simulink model "V4_Modell_komplett"  (R2022a)
settings: Solver=ode3  StartTime=0.0  StopTime=Zeit(end)  FixedStep=0.00001  RelTol=1e-3
values from neighbouring files (symbols this model uses):
  A = 0.01155    [V4_Parameter_Wagen_St.m]    (also in V4_Parameter_Wagen_Te.m; V4_Parameter_komplett_St.m; V4_Parameter_komplett_Te.m)
  c_W = 0.81    [V4_Parameter_Wagen_St.m]    (also in V4_Parameter_Wagen_Te.m; V4_Parameter_komplett_St.m; V4_Parameter_komplett_Te.m)
  g = 9.81    [V4_Parameter_Wagen_St.m]    (also in V4_Parameter_Wagen_Te.m; V4_Parameter_komplett_St.m; V4_Parameter_komplett_Te.m)
  gamma_rad = gamma_deg * (pi/180)    (= 0.349065850399)    [V4_Parameter_Wagen_St.m]    (also in V4_Parameter_Wagen_Te.m; V4_Parameter_komplett_St.m; V4_Parameter_komplett_Te.m)
  k = (m_Trans + m_ErsatzAntrieb + m_ErsatzRad) / (m_Trans)    [V4_Parameter_Wagen_St.m]    (also in V4_Parameter_Wagen_Te.m; V4_Parameter_komplett_St.m; V4_Parameter_komplett_Te.m)
  k_M = -0.038462    [V4_Parameter_EM.m]    (also in V4_Parameter_Wagen_St.m; V4_Parameter_Wagen_Te.m; V4_Parameter_komplett_St.m; V4_Parameter_komplett_Te.m)
  KL_R_VH = [10      20      30      40 ... (first row only)    [V4_Parameter_EM.m]    (also in V4_Parameter_komplett_St.m; V4_Parameter_komplett_Te.m)
  L_A = 0.11 * (10^(-3))    (= 0.00011)    [V4_Parameter_EM.m]    (also in V4_Parameter_komplett_St.m; V4_Parameter_komplett_Te.m)
  m_Trans = m_W + 4*m_R    (= 2.157)    [V4_Parameter_Wagen_St.m]    (also in V4_Parameter_Wagen_Te.m = 1.7232; V4_Parameter_komplett_St.m; V4_Parameter_komplett_Te.m = 1.7232)
  mu_R = 0.043    [V4_Parameter_Wagen_St.m]    (also in V4_Parameter_Wagen_Te.m = 0.045; V4_Parameter_komplett_St.m; V4_Parameter_komplett_Te.m = 0.045)
  R_A = 0.36    [V4_Parameter_EM.m]    (also in V4_Parameter_komplett_St.m; V4_Parameter_komplett_Te.m)
  r_ZR = 25 * (10^(-3))    (= 0.025)    [V4_Parameter_EM.m]    (also in V4_Parameter_Wagen_St.m = 0.021; V4_Parameter_Wagen_Te.m = 0.021; V4_Parameter_komplett_St.m; V4_Parameter_komplett_Te.m)
  rho_L = 1.2    [V4_Parameter_Wagen_St.m]    (also in V4_Parameter_Wagen_Te.m; V4_Parameter_komplett_St.m; V4_Parameter_komplett_Te.m)
undefined symbols (not defined in the file or in its folder): v_rot, x_rot
settings Model: Creator=bornk  LastModifiedBy=bornk

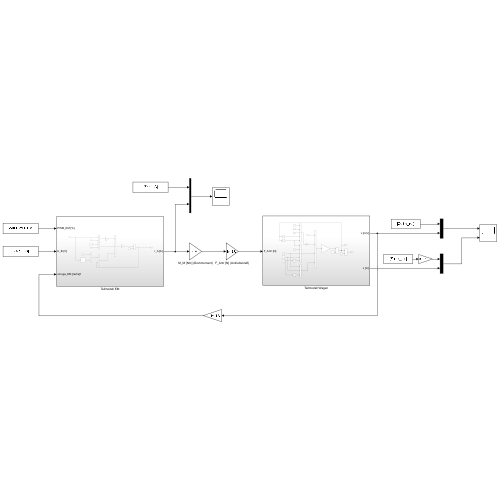
[thumbnail: Simulink's stored preview of the top-level diagram]
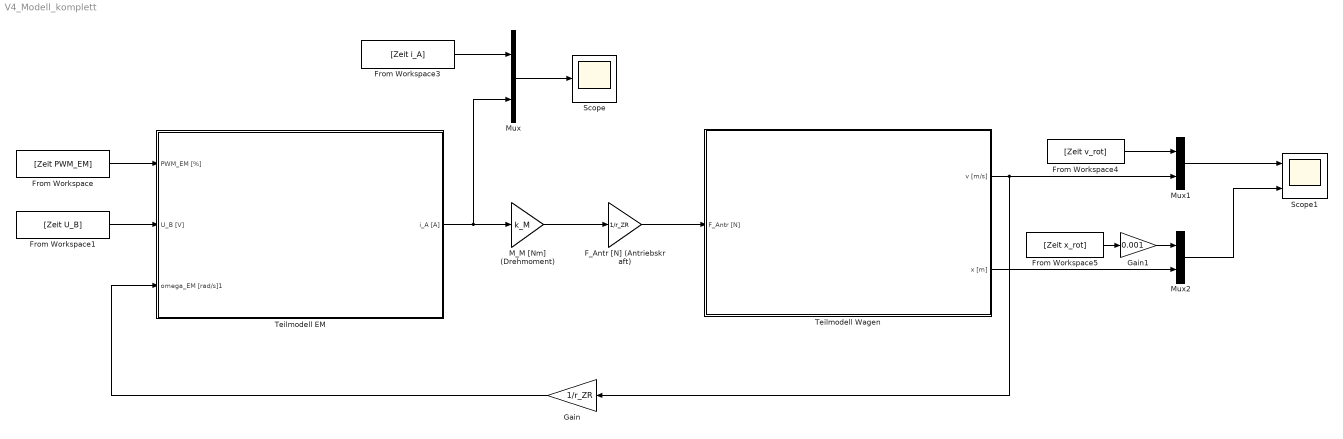
== system V4_Modell_komplett ==
  F_Antr [N] (Antriebskraft) : Gain  Gain=1/r_ZR
  From Workspace : FromWorkspace  VariableName=[Zeit PWM_EM]
  From Workspace1 : FromWorkspace  VariableName=[Zeit U_B]
  From Workspace3 : FromWorkspace  VariableName=[Zeit i_A]
  From Workspace4 : FromWorkspace  VariableName=[Zeit v_rot]
  From Workspace5 : FromWorkspace  VariableName=[Zeit x_rot]
  Gain : Gain  Gain=1/r_ZR
  Gain1 : Gain  Gain=0.001
  M_M [Nm] (Drehmoment) : Gain  Gain=k_M
  Mux : Mux  Inputs=2
  Mux1 : Mux  Inputs=2
  Mux2 : Mux  Inputs=2
  Scope : Scope
  Scope1 : Scope  NumInputPorts=2
  Teilmodell EM : Subsystem
  Teilmodell Wagen : Subsystem
  wires:
  From Workspace1/1 -> Teilmodell EM/2(U_B [V])
  From Workspace3/1 -> Mux/1
  Mux/1 -> Scope/1
  From Workspace/1 -> Teilmodell EM/1(PWM_EM [%])
  From Workspace5/1 -> Gain1/1
  From Workspace4/1 -> Mux1/1
  Mux1/1 -> Scope1/1
  F_Antr [N] (Antriebskraft)/1 -> Teilmodell Wagen/1(F_Antr [N])
  M_M [Nm] (Drehmoment)/1 -> F_Antr [N] (Antriebskraft)/1
  Teilmodell EM/1(i_A [A]) -> Mux/2, M_M [Nm] (Drehmoment)/1
  Gain/1 -> Teilmodell EM/3(omega_EM [rad/s]1)
  Teilmodell Wagen/1(v [m/s]) -> Gain/1, Mux1/2
  Gain1/1 -> Mux2/1
  Teilmodell Wagen/2(x [m]) -> Mux2/2
  Mux2/1 -> Scope1/2

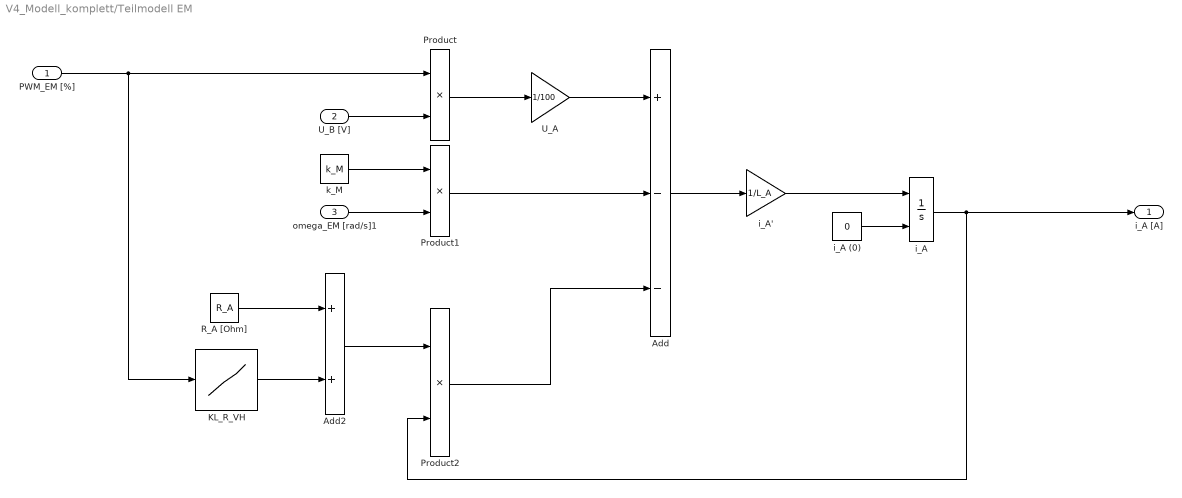
== system V4_Modell_komplett/Teilmodell EM ==
  PWM_EM [%] : Inport
  U_B [V] : Inport  Port=2
  omega_EM [rad/s]1 : Inport  Port=3
  Add : Sum  Inputs=+--
  Add2 : Sum
  KL_R_VH : Lookup_n-D  NumberOfTableDimensions=1  BreakpointsForDimension1=KL_R_VH(1,:)  Table=KL_R_VH(2,:)  InternalRulePriority=Speed  RndMeth=Simplest
  Product : Product
  Product1 : Product
  Product2 : Product
  R_A [Ohm] : Constant  Value=R_A
  U_A : Gain  Gain=1/100
  i_A : Integrator  InitialConditionSource=external
  i_A (0) : Constant  Value=0
  i_A' : Gain  Gain=1/L_A
  k_M : Constant  Value=k_M
  i_A [A] : Outport
  wires:
  i_A'/1 -> i_A/1
  i_A (0)/1 -> i_A/2
  i_A/1 -> Product2/2, i_A [A]/1
  Add/1 -> i_A'/1
  Product/1 -> U_A/1
  U_A/1 -> Add/1
  PWM_EM [%]/1 -> KL_R_VH/1, Product/1
  U_B [V]/1 -> Product/2
  Product1/1 -> Add/2
  omega_EM [rad/s]1/1 -> Product1/2
  k_M/1 -> Product1/1
  Product2/1 -> Add/3
  Add2/1 -> Product2/1
  R_A [Ohm]/1 -> Add2/1
  KL_R_VH/1 -> Add2/2

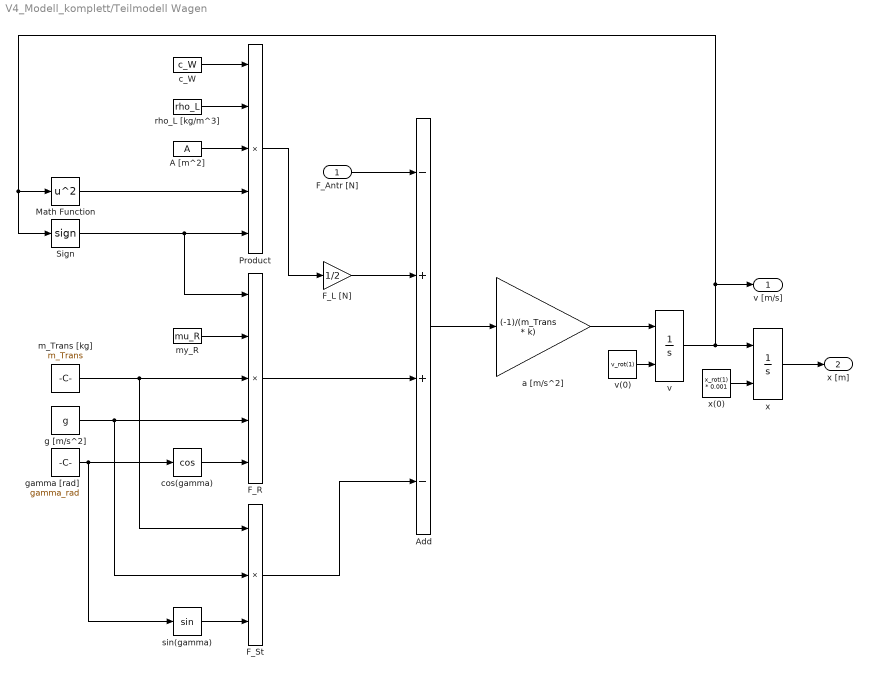
== system V4_Modell_komplett/Teilmodell Wagen ==
  F_Antr [N] : Inport
  A [m^2] : Constant  Value=A
  Add : Sum  Inputs=-++-
  F_L [N] : Gain  Gain=1/2
  F_R : Product  Inputs=5
  F_St : Product  Inputs=3
  Math Function : Math  Operator=square
  Product : Product  Inputs=5
  Sign : Signum
  a [m/s^2] : Gain  Gain=(-1)/(m_Trans * k)
  c_W : Constant  Value=c_W
  cos(gamma) : Trigonometry  Operator=cos
  g [m/s^2] : Constant  Value=g
  gamma [rad] : Constant  Value=gamma_rad
  m_Trans [kg] : Constant  Value=m_Trans
  my_R : Constant  Value=mu_R
  rho_L [kg/m^3] : Constant  Value=rho_L
  sin(gamma) : Trigonometry
  v : Integrator  InitialConditionSource=external
  v(0) : Constant  Value=v_rot(1)
  x : Integrator  InitialConditionSource=external
  x(0) : Constant  Value=x_rot(1) * 0.001
  v [m/s] : Outport
  x [m] : Outport  Port=2
  wires:
  F_Antr [N]/1 -> Add/1
  F_L [N]/1 -> Add/2
  Product/1 -> F_L [N]/1
  A [m^2]/1 -> Product/3
  rho_L [kg/m^3]/1 -> Product/2
  c_W/1 -> Product/1
  Sign/1 -> F_R/1, Product/5
  Math Function/1 -> Product/4
  F_R/1 -> Add/3
  my_R/1 -> F_R/2
  m_Trans [kg]/1 -> F_St/1, F_R/3
  g [m/s^2]/1 -> F_St/2, F_R/4
  gamma [rad]/1 -> sin(gamma)/1, cos(gamma)/1
  cos(gamma)/1 -> F_R/5
  sin(gamma)/1 -> F_St/3
  F_St/1 -> Add/4
  Add/1 -> a [m/s^2]/1
  a [m/s^2]/1 -> v/1
  v(0)/1 -> v/2
  v/1 -> v [m/s]/1, Math Function/1, Sign/1, x/1
  x(0)/1 -> x/2
  x/1 -> x [m]/1
